simulink model "V2x_TC_CarBreakdownWarning_cs"  (Simulink 7.6)
settings: Solver=ode5  SolverMode=SingleTasking  StartTime=0.0  StopTime=18  FixedStep=1/100  RelTol=1e-3
model workspace (MAT data in the model file):
  mbox_table : struct (value not decoded)
  model_closed = 0
  sim_status = 0
PreLoadFcn:
  | check_NUTS_defined;
  | 
  | assignin('base',['model_closed_' bdroot],false);addpath('../includes_V2x');
InitFcn:
  | PreScanExperimentInitFcn(bdroot)
StopFcn:
  | PreScanExperimentStopFcn(bdroot)
undefined symbols (not defined in the file or in its folder): acceleration, actorID, actorType, DiscIntNeverNeededParam, GPS_alt, GPS_lat, GPS_long, intmax, lightBarInUse, messageID, Newton, publicActorType, Raphson, rotZ, sigbuilder_block, sireneInUse, trafficLightPriority, turnAdvice, velocity, x_ini_VRML, y_ini_VRML, yawRate, z_ini_VRML
libraries: simulink x61, PreScanSimulinkLibrary x19, PreScanUsefulBlocks x7, simulink_extras x1
(part 1 of 10)
CloseFcn:
  | evalin('base',['clear model_closed_' bdroot]);
  | 
  | try
  |     close (V2x_TC_GUI)
  | end
  | 
  | try
  |     close (V2X_PlotSpeed)
  | end
settings Model: Creator=PRESCAN  LastModifiedBy=buildbot
settings OptimizationCC: InitFltsAndDblsToZero=on
settings DebuggingCC: SaveWithParameterizedLinksMsg=none  SignalResolutionControl=TryResolveAllWithWarning  SolverPrmCheckMsg=none  MultiTaskDSMMsg=warning  MultiTaskCondExecSysMsg=none
settings SFSimCC: SimParseCustomCode=off
settings RTWCC: IncludeERTFirstTime=on
settings GRTTargetCC: TargetFcnLib=ansi_tfl_tmw.mat

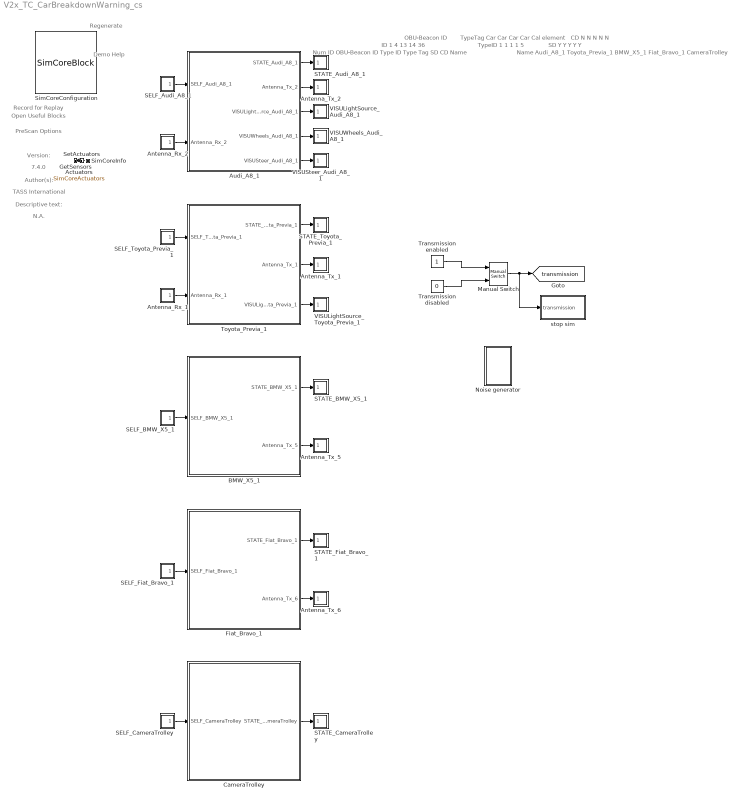
== system V2x_TC_CarBreakdownWarning_cs ==
  note: Demo Help
  note: Regenerate
  note: Record for Replay
  note: Open Useful Blocks
  note: PreScan Options
  note: Version:
  note: 7.4.0
  note: Author(s):
  note: TASS International
  note: Descriptive text:
  note: N.A.
  note: ID
      |
      | 1
      | 4
      | 13
      | 14
      | 36
  note: OBU-Beacon ID
  note: TypeID
      |
      | 1
      | 1
      | 1
      | 1
      | 5
  note: TypeTag
      |
      | Car
      | Car
      | Car
      | Car
      | Cal element
  note: SD
      |
      | Y
      | Y
      | Y
      | Y
      | Y
  note: CD
      |
      | N
      | N
      | N
      | N
      | N
  note: Name
      |
      | Audi_A8_1
      | Toyota_Previa_1
      | BMW_X5_1
      | Fiat_Bravo_1
      | CameraTrolley
  note: Num ID OBU-Beacon ID Type ID Type Tag SD CD Name
  Actuators : DataStoreMemory  Tag=Actuators  DataStoreName=SimCoreActuators  InitialValue=zeros(1299,1)
      settings: DeleteFcn=PreScanBlockDeleteFcn;
  Antenna_Rx_1 : Subsystem  Tag=AntennaR  Priority=3  mask(PreScan Source Block: Antenna Receiver){Channel=1, NrEntitiesOut=3, PortName=Antenna_Rx_1, PortIndex=700, PortWidth=684, TimeStep=1/100}
      mask prompts: Channel "User Specified: Channel# [-]"; NrEntitiesOut "User Specified: # of Visible Actors"; PortName "Auto Assigned: Port Name [-]"; PortIndex "Auto Assigned: Index [-]"; PortWidth "Auto Assigned: Port Dimensions [-]"; TimeStep "Auto Assigned: Upload Period [s]"
      mask help:
      | Using the Antenna Receiver (RX) and Transmitter (TX) information between actors can be exchanged. This is done over a channel number to be specified by the user.
      |
      | The Antenna Reciever receives actor information and user-definable signals.
      |
      | For more information, please click Help.
      settings: DeleteFcn=PreScanBlockDeleteFcn;
      mask Help: eval('openHelp(424)')
      mask Display: image(imread('Rx.png'))
  Antenna_Rx_2 : Subsystem  Tag=AntennaR  Priority=3  mask(PreScan Source Block: Antenna Receiver){Channel=1, NrEntitiesOut=3, PortName=Antenna_Rx_2, PortIndex=8, PortWidth=684, TimeStep=1/100}
      mask prompts: Channel "User Specified: Channel# [-]"; NrEntitiesOut "User Specified: # of Visible Actors"; PortName "Auto Assigned: Port Name [-]"; PortIndex "Auto Assigned: Index [-]"; PortWidth "Auto Assigned: Port Dimensions [-]"; TimeStep "Auto Assigned: Upload Period [s]"
      mask help:
      | Using the Antenna Receiver (RX) and Transmitter (TX) information between actors can be exchanged. This is done over a channel number to be specified by the user.
      |
      | The Antenna Reciever receives actor information and user-definable signals.
      |
      | For more information, please click Help.
      settings: DeleteFcn=PreScanBlockDeleteFcn;
      mask Help: eval('openHelp(424)')
      mask Display: image(imread('Rx.png'))
  Antenna_Tx_1 : Subsystem  Tag=AntennaT  Priority=0  mask(PreScan Sink Block: AntennaT){Channel=1, PortName=Antenna_Tx_1, PortIndex=463, PortWidth=205, TimeStep=1/100}
      mask prompts: Channel "User Specified: Channel# [-]"; PortName "Auto Assigned: Port Name [-]"; PortIndex "Auto Assigned: Index [-]"; PortWidth "Auto Assigned: Port Dimensions [-]"; TimeStep "Auto Assigned: Upload Period [s]"
      mask help:
      | Using the Antenna Receiver (RX) and Transmitter (TX) information between actors can be exchanged. This is done over a channel number to be specified by the user.
      |
      | The Antenna Transmitter contains the following, user-definable signals:
      |
      | - Warning Signal ID	[-]
      | - Maneuvre ID		[-]
      | - Vehicle Type 		[-]
      | - Braking Capacity	[-]
      | - Vehicle Size		[-]
      | - Spares (1:10)		[-]
      |
      | For more information, please click Help.
      settings: DeleteFcn=PreScanBlockDeleteFcn;
      mask Help: eval('openHelp(424)')
      mask Display: image(imread('Tx.png'))
  Antenna_Tx_2 : Subsystem  Tag=AntennaT  Priority=0  mask(PreScan Sink Block: AntennaT){Channel=1, PortName=Antenna_Tx_2, PortIndex=15, PortWidth=205, TimeStep=1/100}
      mask prompts: Channel "User Specified: Channel# [-]"; PortName "Auto Assigned: Port Name [-]"; PortIndex "Auto Assigned: Index [-]"; PortWidth "Auto Assigned: Port Dimensions [-]"; TimeStep "Auto Assigned: Upload Period [s]"
      mask help:
      | Using the Antenna Receiver (RX) and Transmitter (TX) information between actors can be exchanged. This is done over a channel number to be specified by the user.
      |
      | The Antenna Transmitter contains the following, user-definable signals:
      |
      | - Warning Signal ID	[-]
      | - Maneuvre ID		[-]
      | - Vehicle Type 		[-]
      | - Braking Capacity	[-]
      | - Vehicle Size		[-]
      | - Spares (1:10)		[-]
      |
      | For more information, please click Help.
      settings: DeleteFcn=PreScanBlockDeleteFcn;
      mask Help: eval('openHelp(424)')
      mask Display: image(imread('Tx.png'))
  Antenna_Tx_5 : Subsystem  Tag=AntennaT  Priority=0  mask(PreScan Sink Block: AntennaT){Channel=1, PortName=Antenna_Tx_5, PortIndex=859, PortWidth=205, TimeStep=1/100}
      mask prompts: Channel "User Specified: Channel# [-]"; PortName "Auto Assigned: Port Name [-]"; PortIndex "Auto Assigned: Index [-]"; PortWidth "Auto Assigned: Port Dimensions [-]"; TimeStep "Auto Assigned: Upload Period [s]"
      mask help:
      | Using the Antenna Receiver (RX) and Transmitter (TX) information between actors can be exchanged. This is done over a channel number to be specified by the user.
      |
      | The Antenna Transmitter contains the following, user-definable signals:
      |
      | - Warning Signal ID	[-]
      | - Maneuvre ID		[-]
      | - Vehicle Type 		[-]
      | - Braking Capacity	[-]
      | - Vehicle Size		[-]
      | - Spares (1:10)		[-]
      |
      | For more information, please click Help.
      settings: DeleteFcn=PreScanBlockDeleteFcn;
      mask Help: eval('openHelp(424)')
      mask Display: image(imread('Tx.png'))
  Antenna_Tx_6 : Subsystem  Tag=AntennaT  Priority=0  mask(PreScan Sink Block: AntennaT){Channel=1, PortName=Antenna_Tx_6, PortIndex=1079, PortWidth=205, TimeStep=1/100}
      mask prompts: Channel "User Specified: Channel# [-]"; PortName "Auto Assigned: Port Name [-]"; PortIndex "Auto Assigned: Index [-]"; PortWidth "Auto Assigned: Port Dimensions [-]"; TimeStep "Auto Assigned: Upload Period [s]"
      mask help:
      | Using the Antenna Receiver (RX) and Transmitter (TX) information between actors can be exchanged. This is done over a channel number to be specified by the user.
      |
      | The Antenna Transmitter contains the following, user-definable signals:
      |
      | - Warning Signal ID	[-]
      | - Maneuvre ID		[-]
      | - Vehicle Type 		[-]
      | - Braking Capacity	[-]
      | - Vehicle Size		[-]
      | - Spares (1:10)		[-]
      |
      | For more information, please click Help.
      settings: DeleteFcn=PreScanBlockDeleteFcn;
      mask Help: eval('openHelp(424)')
      mask Display: image(imread('Tx.png'))
  Audi_A8_1 : Subsystem  Tag=WorldObjectSubSystem  InitFcn=UniqueId = '20';
      mask Display: image(imread('Audi_A8.jpg'));color('white');text(0,0,' ID=1\n')
  BMW_X5_1 : Subsystem  Tag=WorldObjectSubSystem  InitFcn=UniqueId = '1915';
      mask Display: image(imread('BMW_X5.jpg'));color('white');text(0,0,' ID=13\n')
  CameraTrolley : Subsystem  Tag=WorldObjectSubSystem  InitFcn=UniqueId = '98';
      mask Display: image(imread('Sphere.jpg'));color('white');text(0,0,' ID=36\n')
  Fiat_Bravo_1 : Subsystem  Tag=WorldObjectSubSystem  InitFcn=|
      | UniqueId = '1653';
      | UniqueId = '1924';
      mask Display: image(imread('Fiat_Bravo.jpg'));color('white');text(0,0,' ID=14\n')
  GetSensors : Subsystem  Tag=GetSensors  Priority=2  mask(PreScan Simulation Core Block){NrOfSensors=1408, TimeStep=1/100}
      mask prompts: NrOfSensors "Number of sensor values"; TimeStep "Timestep [s]"
      mask help:
      | Please do not remove this block from the PreScan compilation sheet,
      | as it contains essential configuration parameters for a PreScan simulation.
      settings: DeleteFcn=PreScanBlockDeleteFcn;
  Manual Switch : simulink/Signal Routing/Manual Switch  SystemSampleTime=-1  sw=1  action=0  varsize=off
  Noise generator : Subsystem
  SELF_Audi_A8_1 : Subsystem  Tag=SELF  Priority=3  mask(PreScan Source Block: SELF){PortName=SELF_Audi_A8_1, PortIndex=0, PortWidth=8, TimeStep=1/100}
      mask prompts: PortName "Auto-Assigned: Port Name [-]"; PortIndex "Auto-Assigned: Port Index [-]"; PortWidth "Auto-Assigned: Port Dimensions"; TimeStep "Auto-Assigned: Upload Period [s]"
      mask help:
      | The SELF port shows (state) information of the actor itself. The outputs are position in the experiment's axis system and the GPS coordinates, and the object's absolute velocity and compass heading.
      |
      | For more information, please click Help.
      settings: DeleteFcn=PreScanBlockDeleteFcn;
      mask Help: eval('openHelp(462)')
      mask Display: image(imread('GPS.png'))
  SELF_BMW_X5_1 : Subsystem  Tag=SELF  Priority=3  mask(PreScan Source Block: SELF){PortName=SELF_BMW_X5_1, PortIndex=1384, PortWidth=8, TimeStep=1/100}
      mask prompts: PortName "Auto-Assigned: Port Name [-]"; PortIndex "Auto-Assigned: Port Index [-]"; PortWidth "Auto-Assigned: Port Dimensions"; TimeStep "Auto-Assigned: Upload Period [s]"
      mask help:
      | The SELF port shows (state) information of the actor itself. The outputs are position in the experiment's axis system and the GPS coordinates, and the object's absolute velocity and compass heading.
      |
      | For more information, please click Help.
      settings: DeleteFcn=PreScanBlockDeleteFcn;
      mask Help: eval('openHelp(462)')
      mask Display: image(imread('GPS.png'))
  SELF_CameraTrolley : Subsystem  Tag=SELF  Priority=3  mask(PreScan Source Block: SELF){PortName=SELF_CameraTrolley, PortIndex=1400, PortWidth=8, TimeStep=1/100}
      mask prompts: PortName "Auto-Assigned: Port Name [-]"; PortIndex "Auto-Assigned: Port Index [-]"; PortWidth "Auto-Assigned: Port Dimensions"; TimeStep "Auto-Assigned: Upload Period [s]"
      mask help:
      | The SELF port shows (state) information of the actor itself. The outputs are position in the experiment's axis system and the GPS coordinates, and the object's absolute velocity and compass heading.
      |
      | For more information, please click Help.
      settings: DeleteFcn=PreScanBlockDeleteFcn;
      mask Help: eval('openHelp(462)')
      mask Display: image(imread('GPS.png'))
  SELF_Fiat_Bravo_1 : Subsystem  Tag=SELF  Priority=3  mask(PreScan Source Block: SELF){PortName=SELF_Fiat_Bravo_1, PortIndex=1392, PortWidth=8, TimeStep=1/100}
      mask prompts: PortName "Auto-Assigned: Port Name [-]"; PortIndex "Auto-Assigned: Port Index [-]"; PortWidth "Auto-Assigned: Port Dimensions"; TimeStep "Auto-Assigned: Upload Period [s]"
      mask help:
      | The SELF port shows (state) information of the actor itself. The outputs are position in the experiment's axis system and the GPS coordinates, and the object's absolute velocity and compass heading.
      |
      | For more information, please click Help.
      settings: DeleteFcn=PreScanBlockDeleteFcn;
      mask Help: eval('openHelp(462)')
      mask Display: image(imread('GPS.png'))
  SELF_Toyota_Previa_1 : Subsystem  Tag=SELF  Priority=3  mask(PreScan Source Block: SELF){PortName=SELF_Toyota_Previa_1, PortIndex=692, PortWidth=8, TimeStep=1/100}
      mask prompts: PortName "Auto-Assigned: Port Name [-]"; PortIndex "Auto-Assigned: Port Index [-]"; PortWidth "Auto-Assigned: Port Dimensions"; TimeStep "Auto-Assigned: Upload Period [s]"
      mask help:
      | The SELF port shows (state) information of the actor itself. The outputs are position in the experiment's axis system and the GPS coordinates, and the object's absolute velocity and compass heading.
      |
      | For more information, please click Help.
      settings: DeleteFcn=PreScanBlockDeleteFcn;
      mask Help: eval('openHelp(462)')
      mask Display: image(imread('GPS.png'))
  STATE_Audi_A8_1 : Subsystem  Tag=State  Priority=0  mask(PreScan Sink Block: State){x0=-2.1430611191891602E-16, y0=-1.75, z0=0.55, Roll0=0, Pitch0=0, Yaw0=0, TimeStep=1/100}
      mask prompts: x0 "Ini x-position VEHICLE wrt GLOBAL axis system [m]"; y0 "Ini y-position VEHICLE wrt GLOBAL axis system [m]"; z0 "Ini z-position VEHICLE wrt GLOBAL axis system [m]"; Roll0 "Ini roll-angle BODY wrt VEHICLE axis system [deg]"; Pitch0 "Ini pitch-angle BODY wrt VEHICLE axis system [deg]"; Yaw0 "Ini yaw-angle VEHICLE wrt GLOBAL axis system [deg]"; TimeStep "Time Step [s]"
      mask help:
      | The Actor State contains a vector signal of size (9x1), containing the following signals:
      |
      | -  Position                  (x,y,z)                                     [m]
      | -  Velocity                  (vx,vy,vz)                               [m/s]
      | -  Angles                    (Roll, Pitch, Yaw)                   [rad]
      |
      | The Actor state is defined in the global axis system.
      | The state is superponed on the Initial position defined in the GUI.
      |
      | For more information, please click Help.
      settings: DeleteFcn=PreScanBlockDeleteFcn;
      mask Help: eval('openHelp(222)')
      mask Display: image(imread('State.png'))
  STATE_BMW_X5_1 : Subsystem  Tag=State  Priority=0  mask(PreScan Sink Block: State){x0=213.02464319747571, y0=61.75000509577896, z0=0.69, Roll0=0, Pitch0=0, Yaw0=180, TimeStep=1/100}
      mask prompts: x0 "Ini x-position VEHICLE wrt GLOBAL axis system [m]"; y0 "Ini y-position VEHICLE wrt GLOBAL axis system [m]"; z0 "Ini z-position VEHICLE wrt GLOBAL axis system [m]"; Roll0 "Ini roll-angle BODY wrt VEHICLE axis system [deg]"; Pitch0 "Ini pitch-angle BODY wrt VEHICLE axis system [deg]"; Yaw0 "Ini yaw-angle VEHICLE wrt GLOBAL axis system [deg]"; TimeStep "Time Step [s]"
      mask help:
      | The Actor State contains a vector signal of size (9x1), containing the following signals:
      |
      | -  Position                  (x,y,z)                                     [m]
      | -  Velocity                  (vx,vy,vz)                               [m/s]
      | -  Angles                    (Roll, Pitch, Yaw)                   [rad]
      |
      | The Actor state is defined in the global axis system.
      | The state is superponed on the Initial position defined in the GUI.
      |
      | For more information, please click Help.
      settings: DeleteFcn=PreScanBlockDeleteFcn;
      mask Help: eval('openHelp(222)')
      mask Display: image(imread('State.png'))
  STATE_CameraTrolley : Subsystem  Tag=State  Priority=0  mask(PreScan Sink Block: State){x0=-2.1430611191891602E-16, y0=-1.75, z0=0, Roll0=0, Pitch0=0, Yaw0=0, TimeStep=1/100}
      mask prompts: x0 "Ini x-position VEHICLE wrt GLOBAL axis system [m]"; y0 "Ini y-position VEHICLE wrt GLOBAL axis system [m]"; z0 "Ini z-position VEHICLE wrt GLOBAL axis system [m]"; Roll0 "Ini roll-angle BODY wrt VEHICLE axis system [deg]"; Pitch0 "Ini pitch-angle BODY wrt VEHICLE axis system [deg]"; Yaw0 "Ini yaw-angle VEHICLE wrt GLOBAL axis system [deg]"; TimeStep "Time Step [s]"
      mask help:
      | The Actor State contains a vector signal of size (9x1), containing the following signals:
      |
      | -  Position                  (x,y,z)                                     [m]
      | -  Velocity                  (vx,vy,vz)                               [m/s]
      | -  Angles                    (Roll, Pitch, Yaw)                   [rad]
      |
      | The Actor state is defined in the global axis system.
      | The state is superponed on the Initial position defined in the GUI.
      |
      | For more information, please click Help.
      settings: DeleteFcn=PreScanBlockDeleteFcn;
      mask Help: eval('openHelp(222)')
      mask Display: image(imread('State.png'))
  STATE_Fiat_Bravo_1 : Subsystem  Tag=State  Priority=0  mask(PreScan Sink Block: State){x0=160, y0=61.75, z0=0.55, Roll0=0, Pitch0=0, Yaw0=180, TimeStep=1/100}
      mask prompts: x0 "Ini x-position VEHICLE wrt GLOBAL axis system [m]"; y0 "Ini y-position VEHICLE wrt GLOBAL axis system [m]"; z0 "Ini z-position VEHICLE wrt GLOBAL axis system [m]"; Roll0 "Ini roll-angle BODY wrt VEHICLE axis system [deg]"; Pitch0 "Ini pitch-angle BODY wrt VEHICLE axis system [deg]"; Yaw0 "Ini yaw-angle VEHICLE wrt GLOBAL axis system [deg]"; TimeStep "Time Step [s]"
      mask help:
      | The Actor State contains a vector signal of size (9x1), containing the following signals:
      |
      | -  Position                  (x,y,z)                                     [m]
      | -  Velocity                  (vx,vy,vz)                               [m/s]
      | -  Angles                    (Roll, Pitch, Yaw)                   [rad]
      |
      | The Actor state is defined in the global axis system.
      | The state is superponed on the Initial position defined in the GUI.
      |
      | For more information, please click Help.
      settings: DeleteFcn=PreScanBlockDeleteFcn;
      mask Help: eval('openHelp(222)')
      mask Display: image(imread('State.png'))
  STATE_Toyota_Previa_1 : Subsystem  Tag=State  Priority=0  mask(PreScan Sink Block: State){x0=146.44679260253906, y0=55.277103424072266, z0=0.71, Roll0=0, Pitch0=0, Yaw0=30, TimeStep=1/100}
      mask prompts: x0 "Ini x-position VEHICLE wrt GLOBAL axis system [m]"; y0 "Ini y-position VEHICLE wrt GLOBAL axis system [m]"; z0 "Ini z-position VEHICLE wrt GLOBAL axis system [m]"; Roll0 "Ini roll-angle BODY wrt VEHICLE axis system [deg]"; Pitch0 "Ini pitch-angle BODY wrt VEHICLE axis system [deg]"; Yaw0 "Ini yaw-angle VEHICLE wrt GLOBAL axis system [deg]"; TimeStep "Time Step [s]"
      mask help:
      | The Actor State contains a vector signal of size (9x1), containing the following signals:
      |
      | -  Position                  (x,y,z)                                     [m]
      | -  Velocity                  (vx,vy,vz)                               [m/s]
      | -  Angles                    (Roll, Pitch, Yaw)                   [rad]
      |
      | The Actor state is defined in the global axis system.
      | The state is superponed on the Initial position defined in the GUI.
      |
      | For more information, please click Help.
      settings: DeleteFcn=PreScanBlockDeleteFcn;
      mask Help: eval('openHelp(222)')
      mask Display: image(imread('State.png'))
  SetActuators : Subsystem  Tag=SetActuators  Priority=1  mask(PreScan Simulation Core Block){TimeStep=1/100, NrOfActuators=1299}
      mask prompts: TimeStep "Timestep [s]"; NrOfActuators "Number of actuator values"
      mask help:
      | Please do not remove this block from the PreScan compilation sheet,
      | as it contains essential configuration parameters for a PreScan simulation.
      settings: DeleteFcn=PreScanBlockDeleteFcn;
  SimCoreConfiguration : M-S-Function  Tag=SimCoreConfiguration  Description=68840A43B63BF8E06D449C5E3879BBCEE4A6B46B0200E817F5D548B3C0F21007  FunctionName=SimCoreBlock  Parameters=ExperimentXML PortsXML SimulationCore HostName CheckStart EnableLog RfR EnableGPUAccel ShowComputationTime  mask(PreScan Simulation Core Configurator){SimulationCore=NUTS, HostName=0, CheckStart=0, prescanversion='7.4.0', EnableLog=off, RfR=0, EnableGPUAccel=off, ShowComputationTime=off}
      mask prompts: SimulationCore "Simulation Core"; HostName "Simulation Host"; CheckStart "Show START Dialog"; prescanversion "PreScan Version"; EnableLog "Create TA Log"; RfR "Record for Replay"; EnableGPUAccel "Enable GPU Acceleration"; ShowComputationTime "Show ComputationTime Scope"
      mask help:
      | Please do not remove this block from the PreScan compilation sheet,
      | as it contains essential configuration parameter for a PreScan simulation.
      mask init:
      | model = bdroot;
      | ExperimentXML = [model(1:end-3) '.pex'];
      | PortsXML = [model '_ports.pcd'];
      settings: DeleteFcn=PreScanBlockDeleteFcn;  ModelCloseFcn=assignin('base',['model_closed_' bdroot],true);
      mask Help: eval('openHelp(812)')
      mask Display: image(imread('prescanlogo.ico'))
  SimCoreInfo : Subsystem  Tag=SimCoreInfo
  Toyota_Previa_1 : Subsystem  Tag=WorldObjectSubSystem  InitFcn=UniqueId = '1816';
      mask Display: image(imread('Toyota_Previa.jpg'));color('white');text(0,0,' ID=4\n')
  Transmission disabled : Constant  Value=0
  Transmission enabled : Constant
  VISULightSource_Audi_A8_1 : Subsystem  Tag=VisuLightSource  Priority=0
      settings: DeleteFcn=PreScanBlockDeleteFcn;
      mask Type: PreScan Sink Block: VisuLightSource
      mask Description:
      | The VisuLightSource block provides a way to animate Light Sources of the indicator, braking, fog and main lights of a vehicle.
      | 
      | For more information, please click Help.
      mask Help: eval('openHelp(223)')
      mask Display: image(imread('RearLight.png'))
  VISULightSource_Toyota_Previa_1 : Subsystem  Tag=VisuLightSource  Priority=0
      settings: DeleteFcn=PreScanBlockDeleteFcn;
      mask Type: PreScan Sink Block: VisuLightSource
      mask Description:
      | The VisuLightSource block provides a way to animate Light Sources of the indicator, braking, fog and main lights of a vehicle.
      | 
      | For more information, please click Help.
      mask Help: eval('openHelp(223)')
      mask Display: image(imread('RearLight.png'))
  VISUSteer_Audi_A8_1 : Subsystem  Tag=VisuSteer  Priority=0
      settings: DeleteFcn=PreScanBlockDeleteFcn;
      mask Type: PreScan Sink Block: VisuSteer
      mask Description:
      | The VisuSteer block provides a way to adapt the orientation of the steering column and steering wheel of a vehicle.
      | 
      | For more information, please click Help.
      mask Help: eval('openHelp(223)')
      mask Display: image(imread('steeringwheel.png'))
  VISUWheels_Audi_A8_1 : Subsystem  Tag=VisuWheels  Priority=0
      settings: DeleteFcn=PreScanBlockDeleteFcn;
      mask Type: PreScan Sink Block: VisuWheels
      mask Description:
      | The VisuWheels block provides a way to animate the wheels of a vehicle, with steering, rotation (because of velocity) and z-displacement.
      | 
      | For more information, please click Help.
      mask Help: eval('openHelp(223)')
      mask Display: image(imread('wheel.png'))
  stop sim : Subsystem
  tag scope: transmission=global
  wires:
  Transmission enabled/1 -> Manual Switch/1
  Transmission disabled/1 -> Manual Switch/2
  Manual Switch/1 -> [transmission], stop sim/1(transmission)
  Audi_A8_1/1(STATE_Audi_A8_1) -> STATE_Audi_A8_1/1(State)
  SELF_Audi_A8_1/1(U) -> Audi_A8_1/1(SELF_Audi_A8_1)
  Antenna_Rx_2/1(U) -> Audi_A8_1/2(Antenna_Rx_2)
  Audi_A8_1/2(Antenna_Tx_2) -> Antenna_Tx_2/1(Y)
  Audi_A8_1/3(VISULightSource_Audi_A8_1) -> VISULightSource_Audi_A8_1/1(Lights)
  Audi_A8_1/4(VISUWheels_Audi_A8_1) -> VISUWheels_Audi_A8_1/1(Wheels)
  Audi_A8_1/5(VISUSteer_Audi_A8_1) -> VISUSteer_Audi_A8_1/1(Steer)
  Toyota_Previa_1/1(STATE_Toyota_Previa_1) -> STATE_Toyota_Previa_1/1(State)
  SELF_Toyota_Previa_1/1(U) -> Toyota_Previa_1/1(SELF_Toyota_Previa_1)
  Antenna_Rx_1/1(U) -> Toyota_Previa_1/2(Antenna_Rx_1)
  Toyota_Previa_1/2(Antenna_Tx_1) -> Antenna_Tx_1/1(Y)
  Toyota_Previa_1/3(VISULightSource_Toyota_Previa_1) -> VISULightSource_Toyota_Previa_1/1(Lights)
  BMW_X5_1/1(STATE_BMW_X5_1) -> STATE_BMW_X5_1/1(State)
  SELF_BMW_X5_1/1(U) -> BMW_X5_1/1(SELF_BMW_X5_1)
  BMW_X5_1/2(Antenna_Tx_5) -> Antenna_Tx_5/1(Y)
  Fiat_Bravo_1/1(STATE_Fiat_Bravo_1) -> STATE_Fiat_Bravo_1/1(State)
  SELF_Fiat_Bravo_1/1(U) -> Fiat_Bravo_1/1(SELF_Fiat_Bravo_1)
  Fiat_Bravo_1/2(Antenna_Tx_6) -> Antenna_Tx_6/1(Y)
  CameraTrolley/1(STATE_CameraTrolley) -> STATE_CameraTrolley/1(State)
  SELF_CameraTrolley/1(U) -> CameraTrolley/1(SELF_CameraTrolley)
  SetActuators/1(dummy) -> GetSensors/1(dummy)

== system V2x_TC_CarBreakdownWarning_cs/Antenna_Rx_1 ==
  Selector : Selector  IndexMode=Zero-based  IndexOptions=Starting index (dialog)  Indices=PortIndex  OutputSizes=PortWidth(1)
  U : Outport
  wires:
  Selector/1 -> U/1
  [SimCoreSensors] -> Selector/1

== system V2x_TC_CarBreakdownWarning_cs/Antenna_Rx_2 ==
  Selector : Selector  IndexMode=Zero-based  IndexOptions=Starting index (dialog)  Indices=PortIndex  OutputSizes=PortWidth(1)
  U : Outport
  wires:
  Selector/1 -> U/1
  [SimCoreSensors] -> Selector/1

== system V2x_TC_CarBreakdownWarning_cs/Antenna_Tx_1 ==
  Y : Inport
  Assignment : Assignment  IndexMode=Zero-based  SampleTime=TimeStep  IndexOptions=Starting index (dialog)  Indices=PortIndex  OutputSizes=[1 1]
  Data Store Read : DataStoreRead  DataStoreName=SimCoreActuators  SampleTime=TimeStep
  Data Store Write : DataStoreWrite  DataStoreName=SimCoreActuators
  wires:
  Assignment/1 -> Data Store Write/1
  Data Store Read/1 -> Assignment/1
  Y/1 -> Assignment/2

== system V2x_TC_CarBreakdownWarning_cs/Antenna_Tx_2 ==
  Y : Inport
  Assignment : Assignment  IndexMode=Zero-based  SampleTime=TimeStep  IndexOptions=Starting index (dialog)  Indices=PortIndex  OutputSizes=[1 1]
  Data Store Read : DataStoreRead  DataStoreName=SimCoreActuators  SampleTime=TimeStep
  Data Store Write : DataStoreWrite  DataStoreName=SimCoreActuators
  wires:
  Assignment/1 -> Data Store Write/1
  Data Store Read/1 -> Assignment/1
  Y/1 -> Assignment/2

== system V2x_TC_CarBreakdownWarning_cs/Antenna_Tx_5 ==
  Y : Inport
  Assignment : Assignment  IndexMode=Zero-based  SampleTime=TimeStep  IndexOptions=Starting index (dialog)  Indices=PortIndex  OutputSizes=[1 1]
  Data Store Read : DataStoreRead  DataStoreName=SimCoreActuators  SampleTime=TimeStep
  Data Store Write : DataStoreWrite  DataStoreName=SimCoreActuators
  wires:
  Assignment/1 -> Data Store Write/1
  Data Store Read/1 -> Assignment/1
  Y/1 -> Assignment/2

== system V2x_TC_CarBreakdownWarning_cs/Antenna_Tx_6 ==
  Y : Inport
  Assignment : Assignment  IndexMode=Zero-based  SampleTime=TimeStep  IndexOptions=Starting index (dialog)  Indices=PortIndex  OutputSizes=[1 1]
  Data Store Read : DataStoreRead  DataStoreName=SimCoreActuators  SampleTime=TimeStep
  Data Store Write : DataStoreWrite  DataStoreName=SimCoreActuators
  wires:
  Assignment/1 -> Data Store Write/1
  Data Store Read/1 -> Assignment/1
  Y/1 -> Assignment/2

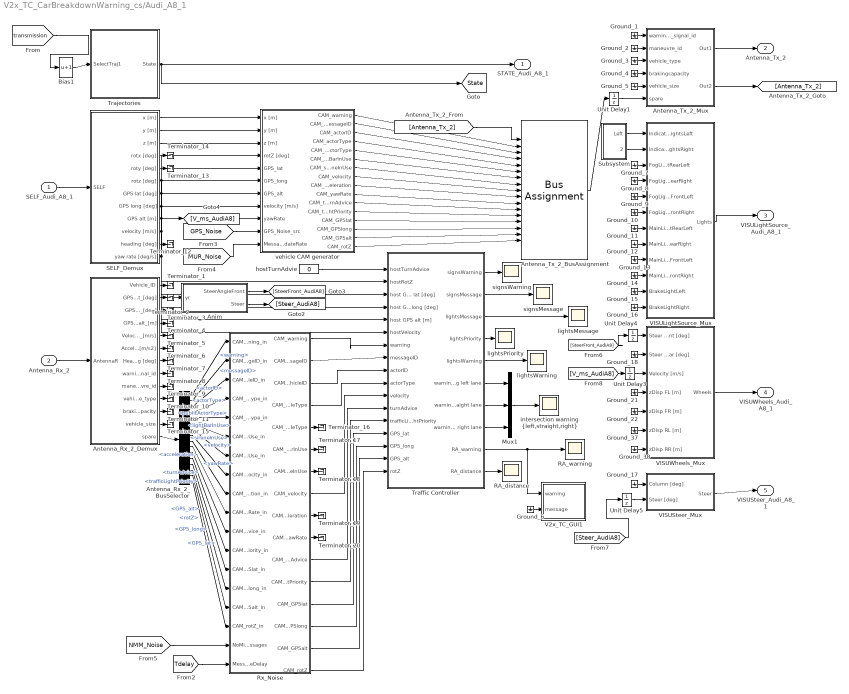
== system V2x_TC_CarBreakdownWarning_cs/Audi_A8_1 ==
  SELF_Audi_A8_1 : Inport  Tag=SELFInport
  Antenna_Rx_2 : Inport  Tag=AntennaRInport  Port=2
  Anim : Subsystem
  Antenna_Rx_2_BusSelector : BusSelector  Tag=BusAntennaR  OutputSignals=warning,messageID,actorID,actorType,publicActorType,lightBarInUse,sireneInUse,velocity,acceleration,yawRate,turnAdvice,trafficLightPriority,GPS_lat,GPS_long,GPS_alt,rotZ
  Antenna_Rx_2_Demux : Subsystem  Tag=DemuxAntennaR  mask(PreScan Demux Block:){Channel=1}
      settings: DeleteFcn=PreScanBlockDeleteFcn;
      mask Display:
      | fprintf('Channel: %d',Channel)
      | port_label('output', 1, 'Vehicle_ID')
      | port_label('output', 2, 'GPS Pos Lat [deg]')
      | port_label('output', 3, 'GPS Pos Long [deg]')
      | port_label('output', 4, 'GPS Pos Alt [m]')
      | port_label('output', 5, 'Velocity [m/s]')
      | port_label('output', 6, 'Acceleration [m/s2]')
      | port_label('output', 7, 'Heading [deg]')
      | port_label('output', 8, 'Warning signal ID')
      | port_label('output', 9, 'Maneuvre ID')
      | port_label('output', 10, 'Vehicle Type')
      | port_label('output', 11, 'Braking Capacity')
      | port_label('output', 12, 'Vehicle Size')
      | port_label('output', 13, 'Spare')
  Antenna_Tx_2_BusAssignment : BusAssignment  Tag=BusAntennaT  AssignedSignals=warning,messageID,actorID,actorType,publicActorType,lightBarInUse,sireneInUse,velocity,acceleration,yawRate,turnAdvice,trafficLightPriority,GPS_lat,GPS_long,GPS_alt,rotZ
  Antenna_Tx_2_Mux : Subsystem  Tag=MuxAntennaT  mask(PreScan Mux Block:){Channel=1, TimeStep=1/100}
      mask prompts: TimeStep "Time Step [s]"
      settings: DeleteFcn=PreScanBlockDeleteFcn;
      mask Display:
      | fprintf('Channel: %d',Channel)
      | port_label('input', 1, 'Warning signal ID')
      | port_label('input', 2, 'Maneuvre ID')
      | port_label('input', 3, 'Vehicle Type')
      | port_label('input', 4, 'Braking Capacity')
      | port_label('input', 5, 'Vehicle Size')
      | port_label('input', 6, 'spare')
  Bias1 : Bias  Bias=1
  Ground_{1..18,21..22,37..38} (22 alike) : Ground
  Mux1 : Mux  Inputs=3
  RA_distance : Scope
      settings: YMin=0  YMax=75  SaveName=ScopeData11
  RA_warning : Scope
      settings: YMin=-0.1  YMax=1.1  SaveName=ScopeData10
  Rx_Noise : Subsystem
  SELF_Demux : Subsystem  Tag=DemuxSELF
      settings: DeleteFcn=PreScanBlockDeleteFcn;
      mask Type: PreScan Demux Block:
      mask Display:
      | port_label('output',1,'x [m]')
      | port_label('output',2,'y [m]')
      | port_label('output',3,'z [m]','texmode','on')
      | port_label('output',4,'Rotx [deg]','texmode','on')
      | port_label('output',5,'Roty [deg]','texmode','on')
      | port_label('output',6,'Rotz [deg]','texmode','on')
      | port_label('output',7,'GPS lat [deg]','texmode','on')
      | port_label('output',8,'GPS long [deg]','texmode','on')
      | port_label('output',9,'GPS alt [m]','texmode','on')
      | port_label('output',10,'Velocity [m/s]')
      | port_label('output',11,'Heading [deg]')
      | port_label('output',12,'Yaw rate [deg/s]')
  Subsystem : Subsystem
  Terminator_{1..20} (20 alike) : Terminator
  Traffic Controller : Subsystem
  Trajectories : Subsystem  Tag=Trajectories
      settings: DeleteFcn=PreScanBlockDeleteFcn;
      mask Type: PreScan Source Block: Trajectories
      mask Description:
      | The Trajectory block contains the trajectories defined in the PreScan Experiment Editor. The output of the trajectory block is the (vehicle) State.
      | 
      | For more information, please click Help.
      mask Help: eval('openHelp(312)')
      mask Display: image(imread('Trajectory.png'));
  Unit Delay{1,3..5} (4 alike) : UnitDelay  SampleTime=-1
  V2x_TC_GUI1 : Subsystem
  VISULightSource_Mux : Subsystem  Tag=MuxLightSource
      settings: DeleteFcn=PreScanBlockDeleteFcn;
      mask Type: PreScan Mux Block:
  VISUSteer_Mux : Subsystem  Tag=MuxSteer
      settings: DeleteFcn=PreScanBlockDeleteFcn;
      mask Type: PreScan Mux Block:
  VISUWheels_Mux : Subsystem  Tag=MuxWheels  mask(PreScan Mux Block:){TimeStep=1/100}
      mask prompts: TimeStep "Auto Assigned: Time Step [s]"
      settings: DeleteFcn=PreScanBlockDeleteFcn;
  hostTurnAdvie : Constant  Value=0
  "intersection warning {left,straight,right}" : Scope
      settings: YMin=-0.1  YMax=1.1  SaveName=ScopeData15
  lightsMessage : Scope
      settings: SaveName=ScopeData14
  lightsPriority : Scope
      settings: SaveName=ScopeData8
  lightsWarning : Scope
      settings: SaveName=ScopeData9
  signsMessage : Scope
      settings: TimeRange=0.1843234764159973  YMin=900.4078101828966  YMax=905.9158957700726  SaveName=ScopeData12
  signsWarning : Scope
      settings: SaveName=ScopeData13
  vehicle CAM generator : Subsystem
  STATE_Audi_A8_1 : Outport  Tag=StateOutport
  Antenna_Tx_2 : Outport  Tag=AntennaTOutport  Port=2
  VISULightSource_Audi_A8_1 : Outport  Tag=VisuLightsOutport  Port=3  SampleTime=1/100
  VISUWheels_Audi_A8_1 : Outport  Tag=VisuWheelsOutport  Port=4  SampleTime=1/100
  VISUSteer_Audi_A8_1 : Outport  Tag=VisuSteerOutport  Port=5  SampleTime=1/100
  tag scope: State=global
  wires:
  hostTurnAdvie/1 -> Traffic Controller/1(hostTurnAdvice)
  Traffic Controller/2(signsMessage) -> signsMessage/1
  Traffic Controller/1(signsWarning) -> signsWarning/1
  Traffic Controller/3(lightsMessage) -> lightsMessage/1
  Traffic Controller/4(lightsPriority) -> lightsPriority/1
  Traffic Controller/5(lightsWarning) -> lightsWarning/1
  Mux1/1 -> "intersection warning {left,straight,right}"/1
  Traffic Controller/6(warning left lane) -> Mux1/1
  Traffic Controller/7(warning straight lane) -> Mux1/2
  Traffic Controller/8(warning right lane) -> Mux1/3
  [NMM_Noise] -> Rx_Noise/17(NoMissedMessages)
  [Tdelay] -> Rx_Noise/18(MessageDelay)
  [GPS_Noise] -> vehicle CAM generator/10(GPS_Noise_src)
  [MUR_Noise] -> vehicle CAM generator/11(MessageUpdateRate)
  Rx_Noise/9(CAM_acceleration) -> Terminator_19/1
  Rx_Noise/10(CAM_yawRate) -> Terminator_20/1
  Rx_Noise/5(CAM_publicVehicleType) -> Terminator_16/1
  Rx_Noise/6(CAM_lightBarInUse) -> Terminator_17/1
  Rx_Noise/7(CAM_sireneInUse) -> Terminator_18/1
  Rx_Noise/1(CAM_warning) -> Traffic Controller/7(warning)
  Rx_Noise/2(CAM_messageID) -> Traffic Controller/8(messageID)
  Rx_Noise/3(CAM_vehicleID) -> Traffic Controller/9(actorID)
  Rx_Noise/4(CAM_vehicleType) -> Traffic Controller/10(actorType)
  Traffic Controller/9(RA_warning) -> RA_warning/1, V2x_TC_GUI1/1(warning)
  Traffic Controller/10(RA_distance) -> RA_distance/1
  Rx_Noise/8(CAM_velocity) -> Traffic Controller/11(velocity)
  Rx_Noise/11(CAM_turnAdvice) -> Traffic Controller/12(turnAdvice)
  Rx_Noise/12(CAM_trafficLightPriority) -> Traffic Controller/13(trafficLightPriority)
  Rx_Noise/13(CAM_GPSlat) -> Traffic Controller/14(GPS_lat)
  Rx_Noise/14(CAM_GPSlong) -> Traffic Controller/15(GPS_long)
  Rx_Noise/15(CAM_GPSalt) -> Traffic Controller/16(GPS_alt)
  Rx_Noise/16(CAM_rotZ) -> Traffic Controller/17(rotZ)
  Anim/2(Steer) -> [Steer_AudiA8]
  Anim/1(SteerAngleFront) -> [SteerFront_AudiA8]
  [transmission] -> Bias1/1
  [V_ms_AudiA8] -> Unit Delay3/1
  [SteerFront_AudiA8] -> Unit Delay4/1
  [Steer_AudiA8] -> Unit Delay5/1
  SELF_Audi_A8_1/1 -> SELF_Demux/1(SELF)
  Antenna_Rx_2_Demux/13(spare) -> Antenna_Rx_2_BusSelector/1
  Antenna_Rx_2/1 -> Antenna_Rx_2_Demux/1(AntennaR)
  Antenna_Tx_2_Mux/2(Out2) -> [Antenna_Tx_2]
  [Antenna_Tx_2] -> Antenna_Tx_2_BusAssignment/1
  Antenna_Tx_2_BusAssignment/1 -> Unit Delay1/1
  Antenna_Tx_2_Mux/1(Out1) -> Antenna_Tx_2/1
  VISULightSource_Mux/1(Lights) -> VISULightSource_Audi_A8_1/1
  VISUWheels_Mux/1(Wheels) -> VISUWheels_Audi_A8_1/1
  VISUSteer_Mux/1(Steer) -> VISUSteer_Audi_A8_1/1
  Trajectories/1(State) -> STATE_Audi_A8_1/1, [State]
  Ground_22/1 -> VISUWheels_Mux/5(zDisp FR [m])
  Ground_21/1 -> VISUWheels_Mux/4(zDisp FL [m])
  Ground_38/1 -> VISUWheels_Mux/7(zDisp RR [m])
  Ground_37/1 -> VISUWheels_Mux/6(zDisp RL [m])
  SELF_Demux/5(roty [deg]) -> Terminator_13/1
  SELF_Demux/4(rotx [deg]) -> Terminator_14/1
  Antenna_Rx_2_Demux/12(vehicle_size) -> Terminator_15/1
  Antenna_Rx_2_BusSelector/16 -> Rx_Noise/16(CAM_rotZ_in)  "<rotZ>"
  Antenna_Rx_2_BusSelector/15 -> Rx_Noise/15(CAM_GPSalt_in)  "<GPS_alt>"
  Antenna_Rx_2_BusSelector/14 -> Rx_Noise/14(CAM_GPSlong_in)  "<GPS_long>"
  Antenna_Rx_2_BusSelector/13 -> Rx_Noise/13(CAM_GPSlat_in)  "<GPS_lat>"
  Antenna_Rx_2_BusSelector/12 -> Rx_Noise/12(CAM_trafficLightPriority_in)  "<trafficLightPriority>"
  Antenna_Rx_2_BusSelector/11 -> Rx_Noise/11(CAM_turnAdvice_in)  "<turnAdvice>"
  Antenna_Rx_2_BusSelector/10 -> Rx_Noise/10(CAM_yawRate_in)  "<yawRate>"
  Antenna_Rx_2_BusSelector/9 -> Rx_Noise/9(CAM_acceleration_in)  "<acceleration>"
  Antenna_Rx_2_BusSelector/8 -> Rx_Noise/8(CAM_velocity_in)  "<velocity>"
  Antenna_Rx_2_BusSelector/7 -> Rx_Noise/7(CAM_sireneInUse_in)  "<sireneInUse>"
  Antenna_Rx_2_BusSelector/6 -> Rx_Noise/6(CAM_lightBarInUse_in)  "<lightBarInUse>"
  Antenna_Rx_2_BusSelector/5 -> Rx_Noise/5(CAM_publicVehicleType_in)  "<publicActorType>"
  Antenna_Rx_2_BusSelector/4 -> Rx_Noise/4(CAM_vehicleType_in)  "<actorType>"
  Antenna_Rx_2_BusSelector/3 -> Rx_Noise/3(CAM_vehicleID_in)  "<actorID>"
  Antenna_Rx_2_BusSelector/2 -> Rx_Noise/2(CAM_messageID_in)  "<messageID>"
  Antenna_Rx_2_BusSelector/1 -> Rx_Noise/1(CAM_warning_in)  "<warning>"
  vehicle CAM generator/16(CAM_rotZ) -> Antenna_Tx_2_BusAssignment/17
  vehicle CAM generator/15(CAM_GPSalt) -> Antenna_Tx_2_BusAssignment/16
  vehicle CAM generator/14(CAM_GPSlong) -> Antenna_Tx_2_BusAssignment/15
  vehicle CAM generator/13(CAM_GPSlat) -> Antenna_Tx_2_BusAssignment/14
  vehicle CAM generator/12(CAM_trafficLightPriority) -> Antenna_Tx_2_BusAssignment/13
  vehicle CAM generator/11(CAM_turnAdvice) -> Antenna_Tx_2_BusAssignment/12
  SELF_Demux/10(velocity [m/s]) -> Traffic Controller/6(hostVelocity), vehicle CAM generator/8(velocity [m/s]), [V_ms_AudiA8]
  SELF_Demux/9(GPS alt [m]) -> vehicle CAM generator/7(GPS_alt), Traffic Controller/5(host GPS alt [m])
  SELF_Demux/8(GPS long [deg]) -> vehicle CAM generator/6(GPS_long), Traffic Controller/4(host GPS long [deg])
  SELF_Demux/7(GPS lat [deg]) -> vehicle CAM generator/5(GPS_lat), Traffic Controller/3(host GPS lat [deg])
  SELF_Demux/1(x [m]) -> vehicle CAM generator/1(x [m])
  SELF_Demux/12(yaw rate [deg/s]) -> vehicle CAM generator/9(yawRate), Anim/1(yr)
  SELF_Demux/3(z [m]) -> vehicle CAM generator/3(z [m])
  SELF_Demux/2(y [m]) -> vehicle CAM generator/2(y [m])
  SELF_Demux/6(rotz [deg]) -> vehicle CAM generator/4(rotZ [deg]), Traffic Controller/2(hostRotZ)
  vehicle CAM generator/1(CAM_warning) -> Antenna_Tx_2_BusAssignment/2
  vehicle CAM generator/2(CAM_messageID) -> Antenna_Tx_2_BusAssignment/3
  vehicle CAM generator/3(CAM_actorID) -> Antenna_Tx_2_BusAssignment/4
  vehicle CAM generator/4(CAM_actorType) -> Antenna_Tx_2_BusAssignment/5
  vehicle CAM generator/5(CAM_publicActorType) -> Antenna_Tx_2_BusAssignment/6
  vehicle CAM generator/6(CAM_lightBarInUse) -> Antenna_Tx_2_BusAssignment/7
  vehicle CAM generator/7(CAM_sireneInUse) -> Antenna_Tx_2_BusAssignment/8
  vehicle CAM generator/8(CAM_velocity) -> Antenna_Tx_2_BusAssignment/9
  vehicle CAM generator/9(CAM_acceleration) -> Antenna_Tx_2_BusAssignment/10
  vehicle CAM generator/10(CAM_yawRate) -> Antenna_Tx_2_BusAssignment/11
  Subsystem/1(Left) -> VISULightSource_Mux/1(IndicatorLightsLeft)
  Subsystem/2(Right) -> VISULightSource_Mux/2(IndicatorLightsRight)
  Unit Delay1/1 -> Antenna_Tx_2_Mux/6(spare)
  Bias1/1 -> Trajectories/1(SelectTraj1)
  Unit Delay3/1 -> VISUWheels_Mux/3(Velocity [m/s])
  Unit Delay4/1 -> VISUWheels_Mux/1(Steer Angle Front [deg])
  Unit Delay5/1 -> VISUSteer_Mux/2(Steer [deg])
  Antenna_Rx_2_Demux/1(Vehicle_ID) -> Terminator_1/1
  Antenna_Rx_2_Demux/2(GPS_pos_lat_[deg]) -> Terminator_2/1
  Antenna_Rx_2_Demux/3(GPS_pos_long_[deg]) -> Terminator_3/1
  Antenna_Rx_2_Demux/4(GPS_pos_alt_[m]) -> Terminator_4/1
  Antenna_Rx_2_Demux/5(Velocity_[m/s]) -> Terminator_5/1
  Antenna_Rx_2_Demux/6(Acceleration_[m/s2]) -> Terminator_6/1
  Antenna_Rx_2_Demux/7(Heading [deg]) -> Terminator_7/1
  Antenna_Rx_2_Demux/8(warning_signal_id) -> Terminator_8/1
  Antenna_Rx_2_Demux/9(maneuvre_id) -> Terminator_9/1
  Antenna_Rx_2_Demux/10(vehicle_type) -> Terminator_10/1
  Antenna_Rx_2_Demux/11(brakingcapacity) -> Terminator_11/1
  Ground_1/1 -> Antenna_Tx_2_Mux/1(warning_signal_id)
  Ground_2/1 -> Antenna_Tx_2_Mux/2(maneuvre_id)
  Ground_3/1 -> Antenna_Tx_2_Mux/3(vehicle_type)
  Ground_4/1 -> Antenna_Tx_2_Mux/4(brakingcapacity)
  Ground_5/1 -> Antenna_Tx_2_Mux/5(vehicle_size)
  SELF_Demux/11(heading [deg]) -> Terminator_12/1
  Ground_6/1 -> V2x_TC_GUI1/2(message)
  Ground_7/1 -> VISULightSource_Mux/3(FogLightRearLeft)
  Ground_8/1 -> VISULightSource_Mux/4(FogLightRearRight)
  Ground_9/1 -> VISULightSource_Mux/5(FogLightFrontLeft)
  Ground_10/1 -> VISULightSource_Mux/6(FogLightFrontRight)
  Ground_11/1 -> VISULightSource_Mux/7(MainLightRearLeft)
  Ground_12/1 -> VISULightSource_Mux/8(MainLightRearRight)
  Ground_13/1 -> VISULightSource_Mux/9(MainLightFrontLeft)
  Ground_14/1 -> VISULightSource_Mux/10(MainLightFrontRight)
  Ground_15/1 -> VISULightSource_Mux/11(BrakeLightLeft)
  Ground_16/1 -> VISULightSource_Mux/12(BrakeLightRight)
  Ground_17/1 -> VISUSteer_Mux/1(Column [deg])
  Ground_18/1 -> VISUWheels_Mux/2(Steer Angle Rear [deg])

== system V2x_TC_CarBreakdownWarning_cs/BMW_X5_1 ==
  SELF_BMW_X5_1 : Inport  Tag=SELFInport
  Antenna_Tx_5_BusAssignment : BusAssignment  Tag=BusAntennaT  AssignedSignals=warning,messageID,actorID,actorType,publicActorType,lightBarInUse,sireneInUse,velocity,acceleration,yawRate,turnAdvice,trafficLightPriority,GPS_lat,GPS_long,GPS_alt,rotZ
  Antenna_Tx_5_Mux : Subsystem  Tag=MuxAntennaT  mask(PreScan Mux Block:){Channel=1, TimeStep=1/100}
      mask prompts: TimeStep "Time Step [s]"
      settings: DeleteFcn=PreScanBlockDeleteFcn;
      mask Display:
      | fprintf('Channel: %d',Channel)
      | port_label('input', 1, 'Warning signal ID')
      | port_label('input', 2, 'Maneuvre ID')
      | port_label('input', 3, 'Vehicle Type')
      | port_label('input', 4, 'Braking Capacity')
      | port_label('input', 5, 'Vehicle Size')
      | port_label('input', 6, 'spare')
  Ground_{1..5} (5 alike) : Ground
  SELF_Demux : Subsystem  Tag=DemuxSELF
      settings: DeleteFcn=PreScanBlockDeleteFcn;
      mask Type: PreScan Demux Block:
      mask Display:
      | port_label('output',1,'x [m]')
      | port_label('output',2,'y [m]')
      | port_label('output',3,'z [m]','texmode','on')
      | port_label('output',4,'Rotx [deg]','texmode','on')
      | port_label('output',5,'Roty [deg]','texmode','on')
      | port_label('output',6,'Rotz [deg]','texmode','on')
      | port_label('output',7,'GPS lat [deg]','texmode','on')
      | port_label('output',8,'GPS long [deg]','texmode','on')
      | port_label('output',9,'GPS alt [m]','texmode','on')
      | port_label('output',10,'Velocity [m/s]')
      | port_label('output',11,'Heading [deg]')
      | port_label('output',12,'Yaw rate [deg/s]')
  Terminator_1 : Terminator
  Terminator_2 : Terminator
  Terminator_3 : Terminator
  Trajectories : Subsystem  Tag=Trajectories
      settings: DeleteFcn=PreScanBlockDeleteFcn;
      mask Type: PreScan Source Block: Trajectories
      mask Description:
      | The Trajectory block contains the trajectories defined in the PreScan Experiment Editor. The output of the trajectory block is the (vehicle) State.
      | 
      | For more information, please click Help.
      mask Help: eval('openHelp(312)')
      mask Display: image(imread('Trajectory.png'));
  Unit Delay : UnitDelay  SampleTime=-1
  vehicle CAM generator : Subsystem
  STATE_BMW_X5_1 : Outport  Tag=StateOutport
  Antenna_Tx_5 : Outport  Tag=AntennaTOutport  Port=2
  wires:
  SELF_BMW_X5_1/1 -> SELF_Demux/1(SELF)
  Antenna_Tx_5_Mux/2(Out2) -> [Antenna_Tx_5]
  [Antenna_Tx_5] -> Antenna_Tx_5_BusAssignment/1
  Antenna_Tx_5_Mux/1(Out1) -> Antenna_Tx_5/1
  Trajectories/1(State) -> STATE_BMW_X5_1/1
  vehicle CAM generator/16(CAM_rotZ) -> Antenna_Tx_5_BusAssignment/17
  vehicle CAM generator/15(CAM_GPSalt) -> Antenna_Tx_5_BusAssignment/16
  vehicle CAM generator/14(CAM_GPSlong) -> Antenna_Tx_5_BusAssignment/15
  vehicle CAM generator/13(CAM_GPSlat) -> Antenna_Tx_5_BusAssignment/14
  vehicle CAM generator/12(CAM_trafficLightPriority) -> Antenna_Tx_5_BusAssignment/13
  vehicle CAM generator/11(CAM_turnAdvice) -> Antenna_Tx_5_BusAssignment/12
  SELF_Demux/12(yaw rate [deg/s]) -> vehicle CAM generator/9(yawRate)
  SELF_Demux/10(velocity [m/s]) -> vehicle CAM generator/8(velocity [m/s])
  SELF_Demux/9(GPS alt [m]) -> vehicle CAM generator/7(GPS_alt)
  SELF_Demux/8(GPS long [deg]) -> vehicle CAM generator/6(GPS_long)
  SELF_Demux/7(GPS lat [deg]) -> vehicle CAM generator/5(GPS_lat)
  SELF_Demux/6(rotz [deg]) -> vehicle CAM generator/4(rotZ [deg])
  SELF_Demux/3(z [m]) -> vehicle CAM generator/3(z [m])
  SELF_Demux/2(y [m]) -> vehicle CAM generator/2(y [m])
  SELF_Demux/1(x [m]) -> vehicle CAM generator/1(x [m])
  vehicle CAM generator/1(CAM_warning) -> Antenna_Tx_5_BusAssignment/2
  vehicle CAM generator/2(CAM_messageID) -> Antenna_Tx_5_BusAssignment/3
  vehicle CAM generator/3(CAM_actorID) -> Antenna_Tx_5_BusAssignment/4
  vehicle CAM generator/4(CAM_actorType) -> Antenna_Tx_5_BusAssignment/5
  vehicle CAM generator/5(CAM_publicActorType) -> Antenna_Tx_5_BusAssignment/6
  vehicle CAM generator/6(CAM_lightBarInUse) -> Antenna_Tx_5_BusAssignment/7
  vehicle CAM generator/7(CAM_sireneInUse) -> Antenna_Tx_5_BusAssignment/8
  vehicle CAM generator/8(CAM_velocity) -> Antenna_Tx_5_BusAssignment/9
  vehicle CAM generator/9(CAM_acceleration) -> Antenna_Tx_5_BusAssignment/10
  vehicle CAM generator/10(CAM_yawRate) -> Antenna_Tx_5_BusAssignment/11
  Unit Delay/1 -> Antenna_Tx_5_Mux/6(spare)
  Antenna_Tx_5_BusAssignment/1 -> Unit Delay/1
  Ground_1/1 -> Antenna_Tx_5_Mux/1(warning_signal_id)
  Ground_2/1 -> Antenna_Tx_5_Mux/2(maneuvre_id)
  Ground_3/1 -> Antenna_Tx_5_Mux/3(vehicle_type)
  Ground_4/1 -> Antenna_Tx_5_Mux/4(brakingcapacity)
  Ground_5/1 -> Antenna_Tx_5_Mux/5(vehicle_size)
  SELF_Demux/4(rotx [deg]) -> Terminator_1/1
  SELF_Demux/5(roty [deg]) -> Terminator_2/1
  SELF_Demux/11(heading [deg]) -> Terminator_3/1

== system V2x_TC_CarBreakdownWarning_cs/CameraTrolley ==
  SELF_CameraTrolley : Inport  Tag=SELFInport
  Demux : Demux  Outputs=[6 1 2]
  Dynamics_Empty : Subsystem  Tag=Dynamics_Empty
      mask Display: port_label('output', 1, 'State');text(0,0,' Empty\n')
  Mux : Mux  Inputs=3
  SELF_Demux : Subsystem  Tag=DemuxSELF
      settings: DeleteFcn=PreScanBlockDeleteFcn;
      mask Type: PreScan Demux Block:
      mask Display:
      | port_label('output',1,'x [m]')
      | port_label('output',2,'y [m]')
      | port_label('output',3,'z [m]','texmode','on')
      | port_label('output',4,'Rotx [deg]','texmode','on')
      | port_label('output',5,'Roty [deg]','texmode','on')
      | port_label('output',6,'Rotz [deg]','texmode','on')
      | port_label('output',7,'GPS lat [deg]','texmode','on')
      | port_label('output',8,'GPS long [deg]','texmode','on')
      | port_label('output',9,'GPS alt [m]','texmode','on')
      | port_label('output',10,'Velocity [m/s]')
      | port_label('output',11,'Heading [deg]')
      | port_label('output',12,'Yaw rate [deg/s]')
  Terminator_{1..13} (13 alike) : Terminator
  STATE_CameraTrolley : Outport  Tag=StateOutport
  wires:
  Demux/1 -> Mux/1
  Demux/2 -> Mux/2
  Demux/3 -> Mux/3
  [State] -> Demux/1
  SELF_CameraTrolley/1 -> SELF_Demux/1(SELF)
  Mux/1 -> STATE_CameraTrolley/1
  Dynamics_Empty/1(State) -> Terminator_1/1
  SELF_Demux/1(x [m]) -> Terminator_2/1
  SELF_Demux/2(y [m]) -> Terminator_3/1
  SELF_Demux/3(z [m]) -> Terminator_4/1
  SELF_Demux/4(rotx [deg]) -> Terminator_5/1
  SELF_Demux/5(roty [deg]) -> Terminator_6/1
  SELF_Demux/6(rotz [deg]) -> Terminator_7/1
  SELF_Demux/7(GPS lat [deg]) -> Terminator_8/1
  SELF_Demux/8(GPS long [deg]) -> Terminator_9/1
  SELF_Demux/9(GPS alt [m]) -> Terminator_10/1
  SELF_Demux/10(velocity [m/s]) -> Terminator_11/1
  SELF_Demux/11(heading [deg]) -> Terminator_12/1
  SELF_Demux/12(yaw rate [deg/s]) -> Terminator_13/1
